simulink model "static_force"  (R2016a)
settings: Solver=FixedStepAuto  StartTime=0.0  StopTime=5  FixedStep=0.1  RelTol=1e-3
libraries: simulink x2
settings Model: Creator=marki  LastModifiedBy=marki

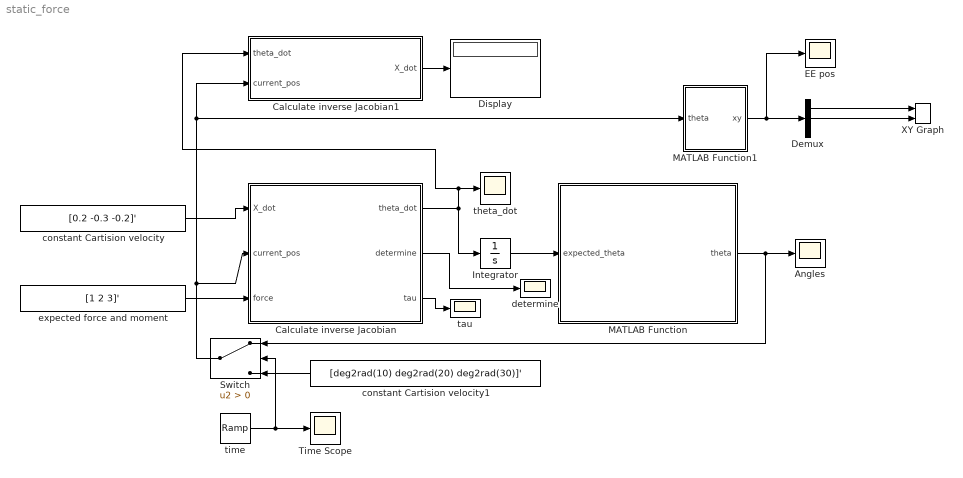
== system static_force ==
  Angles : Scope
  Calculate inverse Jacobian : MATLAB Function  TreatAsAtomicUnit=on
  Calculate inverse Jacobian1 : MATLAB Function  TreatAsAtomicUnit=on
  Demux : Demux  Outputs=3
  Display : Display
  EE pos : Scope
  Integrator : Integrator  InitialCondition=[deg2rad(10) deg2rad(20) deg2rad(30)]'
  MATLAB Function : MATLAB Function  TreatAsAtomicUnit=on
  MATLAB Function1 : MATLAB Function  TreatAsAtomicUnit=on
  Switch : Switch  Criteria=u2 > Threshold
  Time Scope : Scope
  XY Graph : simulink/Sinks/XY Graph  xmin=0  xmax=10  ymin=-5  ymax=5  st=0.1
  constant Cartision velocity : Constant  Value=[0.2 -0.3 -0.2]'
  constant Cartision velocity1 : Constant  Value=[deg2rad(10) deg2rad(20) deg2rad(30)]'
  "determine " : Scope
  expected force and moment : Constant  Value=[1 2 3]'
  tau : Scope
  theta_dot : Scope
  time : simulink/Sources/Ramp  slope=1  start=0  X0=0
  wires:
  Calculate inverse Jacobian/1(theta_dot) -> Integrator/1, Calculate inverse Jacobian1/1(theta_dot), theta_dot/1
  constant Cartision velocity/1 -> Calculate inverse Jacobian/1(X_dot)
  MATLAB Function/1(theta) -> Switch/1, Angles/1
  Switch/1 -> Calculate inverse Jacobian1/2(current_pos), MATLAB Function1/1(theta), Calculate inverse Jacobian/2(current_pos)
  constant Cartision velocity1/1 -> Switch/3
  time/1 -> Time Scope/1, Switch/2
  Integrator/1 -> MATLAB Function/1(expected_theta)
  Demux/1 -> XY Graph/1
  Demux/2 -> XY Graph/2
  MATLAB Function1/1(xy) -> EE pos/1, Demux/1
  Calculate inverse Jacobian1/1(X_dot) -> Display/1
  Calculate inverse Jacobian/2(determine) -> "determine "/1
  expected force and moment/1 -> Calculate inverse Jacobian/3(force)
  Calculate inverse Jacobian/3(tau) -> tau/1

== matlab function static_force/MATLAB Function ==
  data: expected_theta input; theta output
function theta = SCARA_Robot(expected_theta)
%# this is the robot simulator,where output angle is equal to input angle

theta = expected_theta;

== matlab function static_force/Calculate inverse Jacobian ==
  data: X_dot input; current_pos input; theta_dot output; determine output; force input; tau output
function [theta_dot,determine,tau] = inv_Jacobian(X_dot,current_pos,force)
% This function is to calculate the inverse Jacobian
% X_dot represents vector of [x_dot y_dot omega_z]'
%
L1 = 4;
L2 = 3;
L3 = 2;

t1 = current_pos(1);
t2 = current_pos(2);
t3 = current_pos(3);
Jacobian = [-L1*sin(t1)-L2*sin(t1+t2)-L3*sin(t1+t2+t3) -L2*sin(t1+t2)-L3*sin(t1+t2+t3) -L3*sin(t1+t2+t3);
            L1*cos(t1)+L2*cos(t1+t2)+L3*cos(t1+t2+t3)   L2*cos(t1+t2)+L3*cos(t1+t2+t3)  L3*cos(t1+t2+t3);
                            1                                           1                       1       ];
theta_dot = inv(Jacobian)*X_dot;             
determine = det(Jacobian);
tau = Jacobian'*force;

== matlab function static_force/MATLAB Function1 ==
  data: theta input; xy output
function xy = FK(theta)
%# this is the robot simulator,where output angle is equal to input angle
t1 = theta(1);
t2 = theta(2);
t3 = theta(3);
L1=4;
L2 = 3;
L3 = 2;
T01 = [cos(t1) -sin(t1) 0 0;
       sin(t1)  cos(t1) 0 0 ;
        0        0      1 0 ;
        0        0      0 1];
    
T12 = [cos(t2) -sin(t2) 0 L1;
       sin(t2)  cos(t2) 0 0 ;
        0        0      1 0 ;
        0        0      0 1];
    
T23 = [cos(t3) -sin(t3) 0 L2;
       sin(t3)  cos(t3) 0 0 ;
        0        0      1 0 ;
        0        0      0 1];
T3T = [1 0 0 L3;
       0  1 0 0 ;
       0     0      1 0 ;
        0        0      0 1];
    
T_0T = T01*T12*T23*T3T;

R_0T = T_0T(1:3,1:3);


xy = zeros([3 1]);
xy(1) = T_0T(1,4);
xy(2) = T_0T(2,4);
xy(3) = atan2(R_0T(2,1),R_0T(1,1));

== matlab function static_force/Calculate inverse Jacobian1 ==
  data: theta_dot input; current_pos input; X_dot output
function X_dot = Jacobian(theta_dot,current_pos)
% This function is to calculate the inverse Jacobian
% X_dot represents vector of [x_dot y_dot omega_z]'
%
L1 = 4;
L2 = 3;
L3 = 2;

t1 = current_pos(1);
t2 = current_pos(2);
t3 = current_pos(3);
Jacobian = [-L1*sin(t1)-L2*sin(t1+t2)-L3*sin(t1+t2+t3) -L2*sin(t1+t2)-L3*sin(t1+t2+t3) -L3*sin(t1+t2+t3);
            L1*cos(t1)+L2*cos(t1+t2)+L3*cos(t1+t2+t3)   L2*cos(t1+t2)+L3*cos(t1+t2+t3)  L3*cos(t1+t2+t3);
                            1                                           1                       1       ];
X_dot = Jacobian*theta_dot;
